simulink model "LMI"  (R2026b)
settings Model: Creator=Yahoff  LastModifiedBy=Yahoff

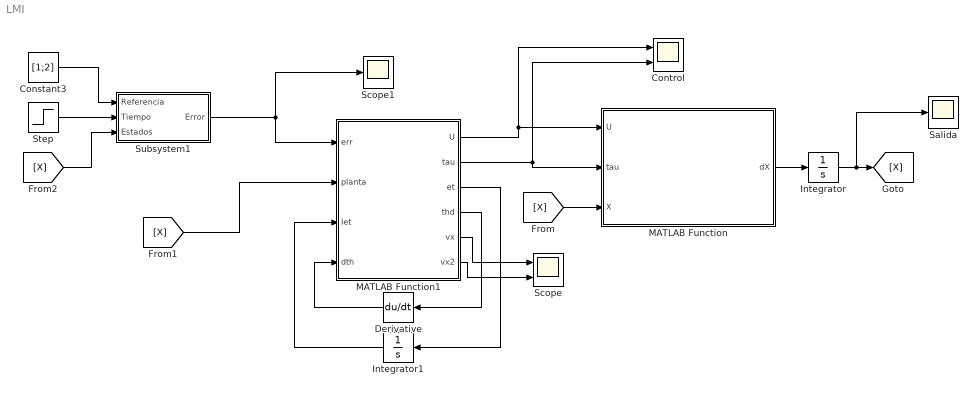
== system LMI ==
  Constant3 : Constant  Value=[1;2]
  Control : Scope  NumInputPorts=2
      settings: ActiveDisplayYMinimum=-282.42325510798588  ActiveDisplayYMaximum=122.76846108803359  DataLoggingVariableName=ScopeData2
  Derivative : Derivative
  Integrator : Integrator  InitialCondition=[0;0;0;0;0;0]
  Integrator1 : Integrator
  MATLAB Function : MATLAB Function  TreatAsAtomicUnit=on
  MATLAB Function1 : MATLAB Function  TreatAsAtomicUnit=on
  Salida : Scope
      settings: ActiveDisplayYMinimum=-0.24908295103818115  ActiveDisplayYMaximum=2.241746559343631
  Scope : Scope  NumInputPorts=2
      settings: ActiveDisplayYMinimum=-3.0769009035102695  ActiveDisplayYMaximum=6.6062096515473749  DataLoggingVariableName=ScopeData3
  Scope1 : Scope
      settings: ActiveDisplayYMinimum=-12610.15580763148  ActiveDisplayYMaximum=4381.1497291038568
  Step : Step  SampleTime=0
  Subsystem1 : Subsystem
  wires:
  MATLAB Function/1(dX) -> Integrator/1
  Integrator/1 -> Salida/1, [X]
  [X] -> MATLAB Function/3(X)
  [X] -> MATLAB Function1/2(planta)
  MATLAB Function1/1(U) -> Control/1, MATLAB Function/1(U)
  MATLAB Function1/2(tau) -> MATLAB Function/2(tau), Control/2
  [X] -> Subsystem1/3(Estados)
  Constant3/1 -> Subsystem1/1(Referencia)
  Step/1 -> Subsystem1/2(Tiempo)
  Subsystem1/1(Error) -> Scope1/1, MATLAB Function1/1(err)
  MATLAB Function1/3(et) -> Integrator1/1
  Derivative/1 -> MATLAB Function1/4(dth)
  MATLAB Function1/4(thd) -> Derivative/1
  Integrator1/1 -> MATLAB Function1/3(Iet)
  MATLAB Function1/5(vx) -> Scope/1
  MATLAB Function1/6(vx2) -> Scope/2

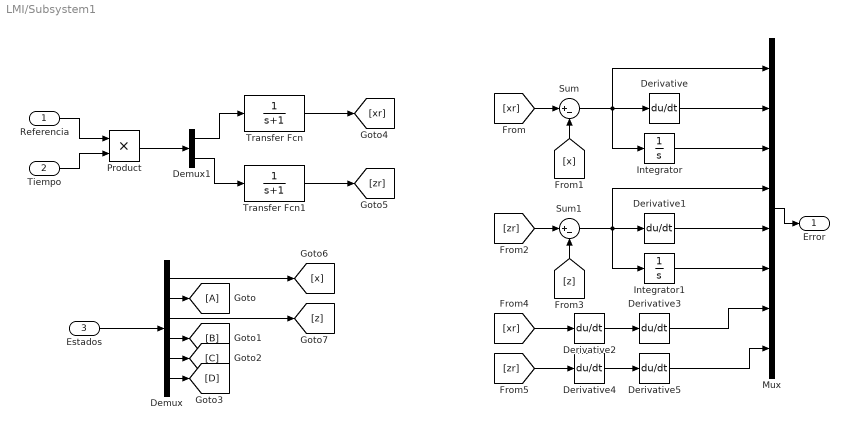
== system LMI/Subsystem1 ==
  Referencia : Inport
  Tiempo : Inport  Port=2
  Estados : Inport  Port=3
  Demux : Demux  Outputs=6
  Demux1 : Demux  Outputs=2
  Derivative{,1..5} (6 alike) : Derivative
  Goto : Goto
  Integrator : Integrator
  Integrator1 : Integrator
  Mux : Mux  Inputs=8
  Product : Product
  Sum : Sum  Inputs=|+-
  Sum1 : Sum  Inputs=|+-
  Transfer Fcn : TransferFcn  Denominator=[1 1]
  Transfer Fcn1 : TransferFcn  Denominator=[1 1]
  Error : Outport
  wires:
  Demux/3 -> [z]
  Demux/1 -> [x]
  Demux/5 -> [C]
  Demux/6 -> [D]
  Estados/1 -> Demux/1
  Demux/2 -> Goto/1
  Demux/4 -> [B]
  Referencia/1 -> Product/1
  Tiempo/1 -> Product/2
  Product/1 -> Demux1/1
  Demux1/2 -> Transfer Fcn1/1
  Demux1/1 -> Transfer Fcn/1
  Transfer Fcn/1 -> [xr]
  Transfer Fcn1/1 -> [zr]
  [xr] -> Sum/1
  [x] -> Sum/2
  [zr] -> Sum1/1
  [z] -> Sum1/2
  Sum/1 -> Derivative/1, Integrator/1, Mux/1
  Sum1/1 -> Derivative1/1, Integrator1/1, Mux/4
  Integrator/1 -> Mux/3
  Integrator1/1 -> Mux/6
  Mux/1 -> Error/1
  Derivative/1 -> Mux/2
  Derivative1/1 -> Mux/5
  [xr] -> Derivative2/1
  Derivative2/1 -> Derivative3/1
  Derivative4/1 -> Derivative5/1
  [zr] -> Derivative4/1
  Derivative3/1 -> Mux/7
  Derivative5/1 -> Mux/8

== matlab function LMI/MATLAB Function1 ==
  data: err input; U output; planta input; tau output; Iet input; et output; dth input; thd output; vx output; vx2 output
function [U, tau,et,thd,vx,vx2] = control(err, planta,Iet,dth)

p = 1; g = 9.81;

K_int = [948.9915 , 40.2834 , 6898.4127]; 
K_x = [17.1814  5.3696  15.6621];   
K_z = K_x;                         

ex  = err(1);
dex = err(2);
Iex = err(3);   
ez  = err(4);
dez = err(5);
Iez = err(6);
xrdd = err(7);
zrdd = err(8);

x     = planta(1);
dx    = planta(2);
z     = planta(3);
dz  = planta(4);
th    = planta(5);
dt = planta(6);

vx = K_x(1)*ex + K_x(2)*dex + K_x(3)*Iex;
vz = K_z(1)*ez + K_z(2)*dez + K_z(3)*Iez;

k=2;%4
m=1;%1
l=2;%2
n=1;%1

sx = dex + n*ex;
vx2 = -n*ex + l*sign(sx);

sz = dez + m*ez;
%vz = -m*ez + k*sign(sz);


U   = p*sqrt(vx^2 + (vz+g)^2);
thd = atan2(-vx, vz+g);

det = dt;

% Lazo interno con LMI
et  = th - thd;
tau = -K_int(1)*et - K_int(2)*det - K_int(3)*Iet;

e = th - thd;
de = dt;

j = 200;
b = 10;

s = de +  b*e;
%tau = - b*de - j*sign(s);

end



function y = sat(u)
if u > 1
    y = 1;
elseif u < -1
    y = -1;
else
    y = u;
end
end

== matlab function LMI/MATLAB Function ==
  data: U input; dX output; tau input; X input
function dX = planta(U, tau, X)

    m = 1; J = 1; g = 9.81;
    kth = 30; kom = 12;

    x     = X(1);
    xdot  = X(2);
    z     = X(3);
    zdot  = X(4);
    th    = X(5);
    thdot = X(6);

    xdd  = -(U/m)*sin(th);
    zdd  =  (U/m)*cos(th) - g;
    thdd =  tau/J;

    dX = [xdot; xdd; zdot; zdd; thdot; thdd];
